simulink model "project_model_O10"  (R2025a)
settings: Solver=FixedStepAuto  StartTime=0.0  StopTime=10.0  FixedStep=1e-3  RelTol=1e-3  EnableMultiTasking=on
undefined symbols (not defined in the file): A0, A1, A2, A3, A4, D0, D10, D11, D12, D13, D2, D3, D4, D5, D6, D7, D8, D9, PTA0, PTA1, PTA2, PTB10, PTB11, PTB2, PTB23, PTB3, PTB9, PTC11, PTC16, PTC2, PTC3, PTC4, PTD0, PTD1, PTD2, PTD3
libraries: frdmk64flib x19
settings Model: ExtModeTrigDuration=5  Creator=justi  LastModifiedBy=justi
settings OptimizationCC: DefaultParameterBehavior=Inlined  EnhancedBackFolding=on  PassReuseOutputArgsAs=Individual arguments  ZeroExternalMemoryAtStartup=off  ZeroInternalMemoryAtStartup=off  MaxStackSize=64  OptimizeBlockOrder=speed  DifferentSizesBufferReuse=on  OptimizationCustomize=off  EfficientTunableParamExpr=on
settings DebuggingCC: ParameterTunabilityLossMsg=error
settings HardwareCC: ProdBitPerPointer=32.0  ProdBitPerSizeT=32.0  ProdBitPerPtrDiffT=32.0  ProdLargestAtomicInteger=Long  ProdLargestAtomicFloat=Double  ProdWordSize=32.0  ProdHWDeviceType=ARM Compatible->ARM Cortex
settings SFSimCC: MATLABDynamicMemAlloc=off
settings RTWCC: SystemTargetFile=ert.tlc  HardwareBoard=NXP FRDM-K64F  TLCOptions="-aInlineSetEventsForThisBaseRateFcn=TLC_FALSE -aSuppressMultiTaskScheduler=TLC_FALSE  -aRateBasedStepFcn=0"  TemplateMakefile=ert_default_tmf  Toolchain=GNU Tools for ARM Embedded Processors  Description=Embedded Coder
settings CodeAppCC: ForceParamTrailComments=on  IgnoreCustomStorageClasses=off  OperatorAnnotations=on  SimulinkDataObjDesc=on  SFDataObjDesc=on  InsertBlockDesc=on
settings ERTTargetCC: ExtModeTransport=4.0  ExtModeStaticAlloc=off  ExtModeMexFile=sendToCommService  ExtModeIntrfLevel=Level1

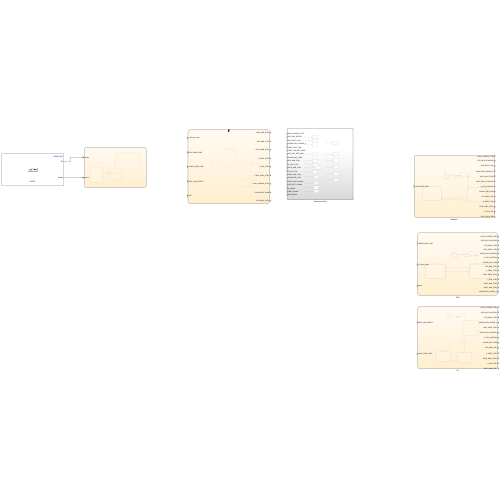
[thumbnail: Simulink's stored preview of the top-level diagram]
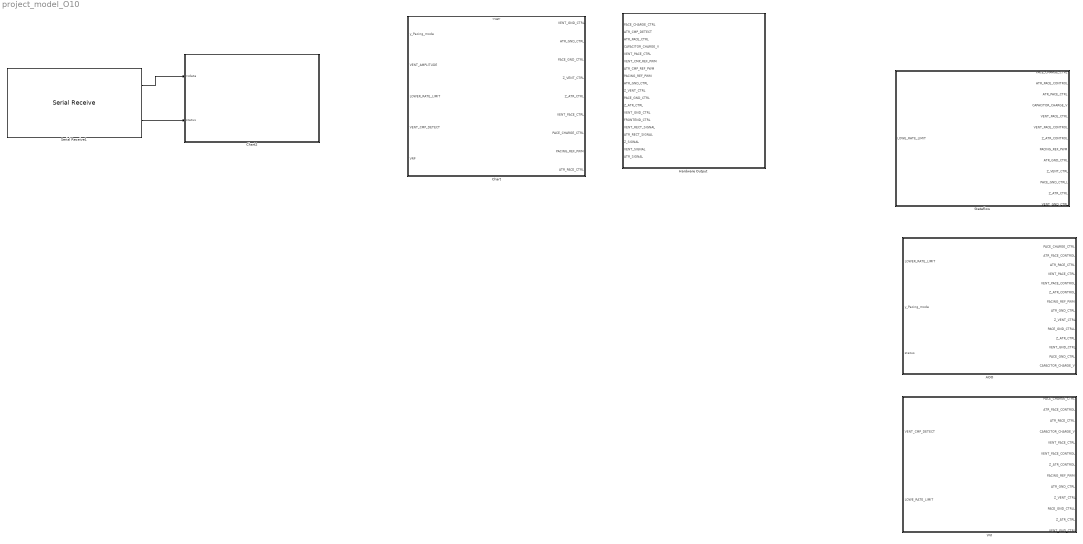
== system project_model_O10 ==
  AOO : Stateflow chart  TreatAsAtomicUnit=on
  Chart : Stateflow chart  TreatAsAtomicUnit=on
  Chart2 : Stateflow chart  TreatAsAtomicUnit=on
  Hardware Output : Subsystem
  Serial Receive1 : frdmk64flib/Serial Receive  SCIModule=0  Baudrate=uint32(9600)  Parity=None  StopBits=1  HardwareFlowControl=None  ByteOrder=LittleEndian  DataType=uint8  DataLength=10  BlockingMode=off  OutputStatus=on  SampleTime=0.1
  "Stateflow " : Stateflow chart  TreatAsAtomicUnit=on
  VVI : Stateflow chart  TreatAsAtomicUnit=on
  wires:
  Serial Receive1/2 -> Chart2/2(status)
  Serial Receive1/1 -> Chart2/1(rxdata)

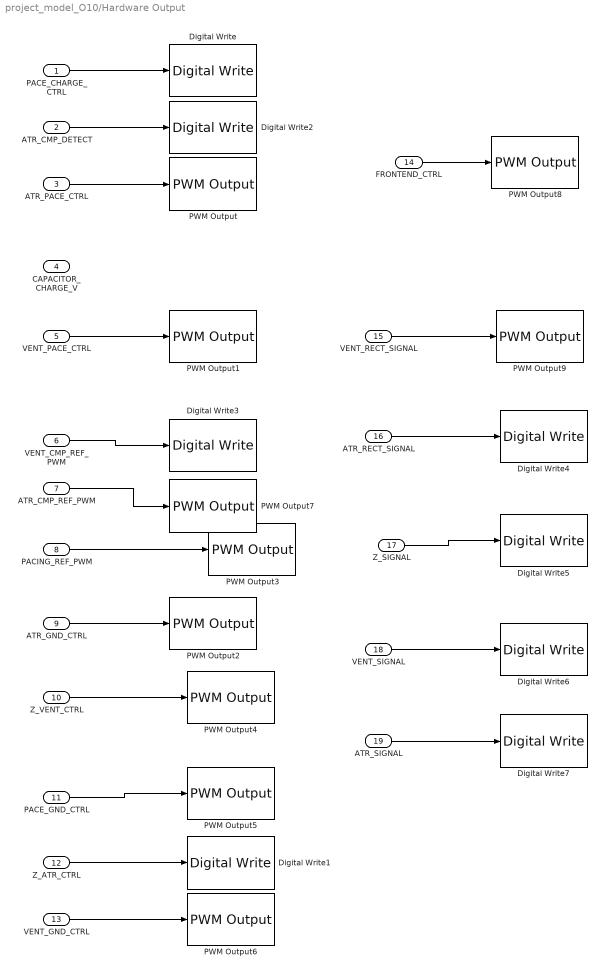
== system project_model_O10/Hardware Output ==
  PACE_CHARGE_CTRL : Inport
  ATR_CMP_DETECT : Inport  Port=2
  ATR_PACE_CTRL : Inport  Port=3
  CAPACITOR_CHARGE_V : Inport  Port=4
  VENT_PACE_CTRL : Inport  Port=5
  VENT_CMP_REF_PWM : Inport  Port=6
  ATR_CMP_REF_PWM : Inport  Port=7
  PACING_REF_PWM : Inport  Port=8
  ATR_GND_CTRL : Inport  Port=9
  Z_VENT_CTRL : Inport  Port=10
  PACE_GND_CTRL : Inport  Port=11
  Z_ATR_CTRL : Inport  Port=12
  VENT_GND_CTRL : Inport  Port=13
  FRONTEND_CTRL : Inport  Port=14
  VENT_RECT_SIGNAL : Inport  Port=15
  ATR_RECT_SIGNAL : Inport  Port=16
  Z_SIGNAL : Inport  Port=17
  VENT_SIGNAL : Inport  Port=18
  ATR_SIGNAL : Inport  Port=19
  Digital Write : frdmk64flib/Digital Write  Whichpin=PTB9 (D2)
  Digital Write1 : frdmk64flib/Digital Write  Whichpin=PTB23 (D4)
  Digital Write2 : frdmk64flib/Digital Write  Whichpin=PTC16 (D0)
  Digital Write3 : frdmk64flib/Digital Write  Whichpin=PTA1 (D3)
  Digital Write4 : frdmk64flib/Digital Write  Whichpin=PTB11 (A3)
  Digital Write5 : frdmk64flib/Digital Write  Whichpin=PTB10 (A2)
  Digital Write6 : frdmk64flib/Digital Write  Whichpin=PTB3 (A1)
  Digital Write7 : frdmk64flib/Digital Write  Whichpin=PTB2 (A0)
  PWM Output : frdmk64flib/PWM Output  Whichpin=PTA0 (D8)  InitialFrequency=2000  InitialDutyCycle=0
  PWM Output1 : frdmk64flib/PWM Output  Whichpin=PTC4 (D9)  InitialFrequency=2000  InitialDutyCycle=0
  PWM Output2 : frdmk64flib/PWM Output  Whichpin=PTD2 (D11)  InitialFrequency=2000  InitialDutyCycle=0
  PWM Output3 : frdmk64flib/PWM Output  Whichpin=PTA2 (D5)  InitialFrequency=2000  InitialDutyCycle=0
  PWM Output4 : frdmk64flib/PWM Output  Whichpin=PTC3 (D7)  InitialFrequency=2000  InitialDutyCycle=0
  PWM Output5 : frdmk64flib/PWM Output  Whichpin=PTD0 (D10)  InitialFrequency=2000  InitialDutyCycle=0
  PWM Output6 : frdmk64flib/PWM Output  Whichpin=PTD3 (D12)  InitialFrequency=2000  InitialDutyCycle=0
  PWM Output7 : frdmk64flib/PWM Output  Whichpin=PTC2 (D6)  InitialFrequency=2000  InitialDutyCycle=0
  PWM Output8 : frdmk64flib/PWM Output  Whichpin=PTD1 (D13)  InitialFrequency=2000  InitialDutyCycle=0
  PWM Output9 : frdmk64flib/PWM Output  Whichpin=PTC11 (A4)  InitialFrequency=2000  InitialDutyCycle=0
  wires:
  PACE_CHARGE_CTRL/1 -> Digital Write/1
  ATR_PACE_CTRL/1 -> PWM Output/1
  VENT_PACE_CTRL/1 -> PWM Output1/1
  ATR_GND_CTRL/1 -> PWM Output2/1
  PACING_REF_PWM/1 -> PWM Output3/1
  Z_VENT_CTRL/1 -> PWM Output4/1
  PACE_GND_CTRL/1 -> PWM Output5/1
  VENT_GND_CTRL/1 -> PWM Output6/1
  Z_ATR_CTRL/1 -> Digital Write1/1
  ATR_CMP_DETECT/1 -> Digital Write2/1
  VENT_CMP_REF_PWM/1 -> Digital Write3/1
  ATR_CMP_REF_PWM/1 -> PWM Output7/1
  FRONTEND_CTRL/1 -> PWM Output8/1
  VENT_RECT_SIGNAL/1 -> PWM Output9/1
  ATR_RECT_SIGNAL/1 -> Digital Write4/1
  Z_SIGNAL/1 -> Digital Write5/1
  VENT_SIGNAL/1 -> Digital Write6/1
  ATR_SIGNAL/1 -> Digital Write7/1

== stateflow chart project_model_O10/VVI ==
  state INITIAL
    entry:
  state STANDBY
  state Initial_Charge_Discharge
    PACE_GND_CTRL=1;
    VENT_PACE_CTRL=0;
    Z_ATR_CTRL=0;
    Z_VENT_CTRL=0;
    ATR_PACE_CTRL=0;
    ATR_GND_CTRL=0;
    VENT_GND_CTRL=1;
    ATR_PACE_CTRL=0;
    VENT_PACE_CTRL=0;
    PACING_REF_PWM=VENT_AMPLITUDE/5000;
    CAPACITOR_CHARGE_V=5;
    PACE_CHARGE_CTRL=1;
    PACE_CHARGE_CTRL=0;
    PACE_GND_CTRL=1;
    ATR_PACE_CTRL=0;
    ATR_GND_CTRL=0;
    Z_ATR_CTRL=0;
    Z_VENT_CTRL=0;
    VENT_GND_CTRL=0;
    VENT_PACE_CTRL=1;
  state Wait_State
  state Discharge
    PACE_CHARGE_CTRL=0;
    PACE_GND_CTRL=1;
    ATR_PACE_CTRL=0;
    ATR_GND_CTRL=0;
    Z_ATR_CTRL=0;
    Z_VENT_CTRL=0;
    VENT_GND_CTRL=0;
    VENT_PACE_CTRL=1;
  state Charge
    PACE_GND_CTRL=1;
    VENT_PACE_CTRL=0;
    Z_ATR_CTRL=0;
    Z_VENT_CTRL=0;
    ATR_PACE_CTRL=0;
    ATR_GND_CTRL=0;
    VENT_GND_CTRL=1;
    ATR_PACE_CTRL=0;
    VENT_PACE_CTRL=0;
    PACING_REF_PWM=VENT_AMPLITUDE/5000;
    CAPACITOR_CHARGE_V=5;
    PACE_CHARGE_CTRL=1;
  (default) -> INITIAL
  (junction 40) -> STANDBY [order 2]
  INITIAL -> STANDBY
  STANDBY -> (junction 40) : [status==0]
  (junction 40) -> Initial_Charge_Discharge [order 1] : [y_Pacing_mode == "VVI"]
  Initial_Charge_Discharge -> Wait_State
  Discharge -> Wait_State
  (junction 64) -> Wait_State [order 1] : [VENT_CMP_DETECT == true]
  Wait_State -> (junction 64) : [after(VRP, mSec)]
  (junction 64) -> Charge [order 2]
  Charge -> Discharge
  data: VENT_CMP_DETECT input; PACE_CHARGE_CTRL output; ATR_PACE_CONTROL output; ATR_PACE_CTRL output; CAPACITOR_CHARGE_V output; VENT_PACE_CTRL output; VENT_PACE_CONTROL output; Z_ATR_CONTROL output; PACING_REF_PWM output; ATR_GND_CTRL output; Z_VENT_CTRL output; PACE_GND_CTRLL output; Z_ATR_CTRL output; VENT_GND_CTRL output; LOWE_RATE_LIMIT input

== stateflow chart project_model_O10/Stateflow  ==
  state INITIAL
    entry:
  state STANDBY
  state Discharge
    PACE_CHARGE_CTRL=0;
    PACE_GND_CTRL=1;
    ATR_PACE_CTRL=0;
    ATR_GND_CTRL=0;
    Z_ATR_CTRL=0;
    Z_VENT_CTRL=0;
    VENT_GND_CTRL=0;
    VENT_PACE_CTRL=1;
  state Charge
    PACE_GND_CTRL=1;
    VENT_PACE_CTRL=0;
    Z_ATR_CTRL=0;
    Z_VENT_CTRL=0;
    ATR_PACE_CTRL=0;
    ATR_GND_CTRL=0;
    VENT_GND_CTRL=1;
    ATR_PACE_CTRL=0;
    VENT_PACE_CTRL=0;
    PACING_REF_PWM=2000;%todo
    CAPACITOR_CHARGE_V=5;
    PACE_CHARGE_CTRL=1;
  (default) -> INITIAL
  (junction 40) -> STANDBY [order 1]
  INITIAL -> STANDBY
  STANDBY -> (junction 40) : [status==0]
  (junction 40) -> Charge [order 2] : [y_Pacing_mode == "VOO"]
  Charge -> Discharge : [after((LOWER_RATE_LIMIT/2),sec)]
  Discharge -> Charge : [after((LOWER_RATE_LIMIT/2),sec)]
  data: PACE_CHARGE_CTRL output; ATR_PACE_CONTROL output; ATR_PACE_CTRL output; CAPACITOR_CHARGE_V output; VENT_PACE_CTRL output; VENT_PACE_CONTROL output; Z_ATR_CONTROL output; PACING_REF_PWM output; ATR_GND_CTRL output; Z_VENT_CTRL output; PACE_GND_CTRLL output; Z_ATR_CTRL output; VENT_GND_CTRL output; LOWE_RATE_LIMIT input

== stateflow chart project_model_O10/Chart ==
  state INITIAL3
    entry:
  state STANDBY3
  state Initial_Pace_VVI
    PACE_GND_CTRL=1;
    VENT_PACE_CTRL=0;
    Z_ATR_CTRL=0;
    Z_VENT_CTRL=0;
    ATR_PACE_CTRL=0;
    ATR_GND_CTRL=0;
    VENT_GND_CTRL=1;
    ATR_PACE_CTRL=0;
    VENT_PACE_CTRL=0;
    PACING_REF_PWM=VENT_AMPLITUDE/5000;
    CAPACITOR_CHARGE_V=5;
    PACE_CHARGE_CTRL=1;
    PACE_CHARGE_CTRL=0;
    PACE_GND_CTRL=1;
    ATR_PACE_CTRL=0;
    ATR_GND_CTRL=0;
    Z_ATR_CTRL=0;
    Z_VENT_CTRL=0;
    VENT_GND_CTRL=0;
    VENT_PACE_CTRL=1;
  state Discharge_VOO
    PACE_CHARGE_CTRL=0;
    PACE_GND_CTRL=1;
    ATR_PACE_CTRL=0;
    ATR_GND_CTRL=0;
    Z_ATR_CTRL=0;
    Z_VENT_CTRL=0;
    VENT_GND_CTRL=0;
    VENT_PACE_CTRL=1;
  state Charge_VOO
    PACE_GND_CTRL=1;
    VENT_PACE_CTRL=0;
    Z_ATR_CTRL=0;
    Z_VENT_CTRL=0;
    ATR_PACE_CTRL=0;
    ATR_GND_CTRL=0;
    VENT_GND_CTRL=1;
    ATR_PACE_CTRL=0;
    VENT_PACE_CTRL=0;
    PACING_REF_PWM=VENT_AMPLITUDE/5000;
    PACE_CHARGE_CTRL=1;
  state Discharge_AOO
    PACE_CHARGE_CTRL=0;
    PACE_GND_CTRL=1;
    VENT_PACE_CTRL=0;
    VENT_GND_CTRL=0;
    Z_VENT_CTRL=0;
    Z_ATR_CTRL=0;
    ATR_GND_CTRL=0;
    ATR_PACE_CTRL=1;
  state Charge_AOO
    PACE_GND_CTRL=1;
    ATR_PACE_CTRL=0;
    Z_VENT_CTRL=0;
    Z_ATR_CTRL=0;
    VENT_PACE_CTRL=0;
    VENT_GND_CTRL=0;
    ATR_GND_CTRL=1;
    VENT_PACE_CTRL=0;
    ATR_PACE_CTRL=0;
    PACING_REF_PWM=2000;%todo
    PACE_CHARGE_CTRL=1;
  state Wait_State
  state Discharge_VVI
    PACE_CHARGE_CTRL=0;
    PACE_GND_CTRL=1;
    ATR_PACE_CTRL=0;
    ATR_GND_CTRL=0;
    Z_ATR_CTRL=0;
    Z_VENT_CTRL=0;
    VENT_GND_CTRL=0;
    VENT_PACE_CTRL=1;
  state Charge_VVI
    PACE_GND_CTRL=1;
    VENT_PACE_CTRL=0;
    Z_ATR_CTRL=0;
    Z_VENT_CTRL=0;
    ATR_PACE_CTRL=0;
    ATR_GND_CTRL=0;
    VENT_GND_CTRL=1;
    ATR_PACE_CTRL=0;
    VENT_PACE_CTRL=0;
    PACING_REF_PWM=VENT_AMPLITUDE/5000;
    CAPACITOR_CHARGE_V=5;
    PACE_CHARGE_CTRL=1;
  (default) -> INITIAL3
  (junction 57) -> STANDBY3 [order 4]
  INITIAL3 -> STANDBY3
  STANDBY3 -> (junction 57) : [status==0]
  (junction 57) -> Initial_Pace_VVI [order 1] : [y_Pacing_mode == "VVI"]
  (junction 57) -> Charge_VOO [order 3] : [y_Pacing_mode == "VOO"]
  (junction 57) -> Charge_AOO [order 2] : [y_Pacing_mode == "AOO"]
  Charge_AOO -> Discharge_AOO : [after((LOWER_RATE_LIMIT/2),mSec)]
  Discharge_AOO -> Charge_AOO : [after((LOWER_RATE_LIMIT/2),mSec)]
  Charge_VOO -> Discharge_VOO : [after((LOWER_RATE_LIMIT/2),mSec)]
  Discharge_VOO -> Charge_VOO : [after((LOWER_RATE_LIMIT/2),mSec)]
  Initial_Pace_VVI -> Wait_State
  Discharge_VVI -> Wait_State
  (junction 28) -> Wait_State [order 1] : [VENT_CMP_DETECT == true]
  Wait_State -> (junction 28) : [after(VRP, mSec)]
  (junction 28) -> Charge_VVI [order 2] : [after(LOWER_RATE_LIMIT-VRP, mSec)]
  Charge_VVI -> Discharge_VVI
  data: y_Pacing_mode input; VENT_GND_CTRL output; ATR_GND_CTRL output; PACE_GND_CTRL output; Z_VENT_CTRL output; Z_ATR_CTRL output; VENT_PACE_CTRL output; PACE_CHARGE_CTRL output; PACING_REF_PWM output; ATR_PACE_CTRL output; VENT_AMPLITUDE input; LOWER_RATE_LIMIT input; VENT_CMP_DETECT input; VRP input
  events: mSec input RISING_EDGE_EVENT

== stateflow chart project_model_O10/Chart2 ==
  state SET_PARAM_
    entry:
    LOWER_RATE_LIMIT=typecast(rxdata(3:4),'uint16');
    UPPER_RATE_LIMIT=typecast(rxdata(5:6),'uint16');
    MAXIMUM_SENSOR_RATE=typecast(rxdata(7:8),'uint16');
    FIXED_AV_DELAY=typecast(rxdata(9:10),'uint16');
    DYNAMIC_AV_DELAY=typecast(rxdata(11:12),'uint16');
    SENSED_AV_DELAY_OFFSET=typecast(rxdata(13:14),'uint16');
    ATRIAL_AMPLITUDE=typecast(rxdata(15:16),'uint16');
    VENTRICULAR_AMPLITUDE=typecast(rxdata(17:18),'uint16');
    ATRIAL_PULSE_WIDTH=typecast(rxdata(19:20),'uint16');
    VENTRICULAR_PULSE_WIDTH=typecast(rxdata(21:22),'uint16');
    ATRIAL_SENSITIVITY=typecast(rxdata(23:24),'uint16');
    VENTRICULAR_SENSITIVITY=typecast(rxdata(25:26),'uint16');
    VRP=typecast(rxdata(27:28),'uint16');
    ARP=typecast(rxdata(29:30),'uint16');
    PVARP=typecast(rxdata(31:32),'uint16');
    PVARP_EXTENSION=typecast(rxdata(33:34),'uint16');
    HYSTERESIS=typecast(rxdata(35:36),'uint16');
    RATE_SMOOTHING=typecast(rxdata(37:38),'uint16');
    ATR_DURATION=typecast(rxdata(39:40),'uint16');
    ATR_FALLBACK_MODE=typecast(rxdata(41:42),'uint16');
    ATR_FALLBACK_TIME=typecast(rxdata(43:44),'uint16');
    ACTIVITY_THRESHOLD=typecast(rxdata(45:46),'uint16');
    REACTION_TIME=typecast(rxdata(47:48),'uint16');
    RESPONSE_FACTOR=typecast(rxdata(49:50),'uint16');
    RECOVERY_TIME=typecast(rxdata(51:52),'uint16');
  state INITIAL
    entry:
    LOWER_RATE_LIMIT = 0;
    UPPER_RATE_LIMIT = 0;
    MAXIMUM_SENSOR_RATE = 0;
    FIXED_AV_DELAY = 0;
    DYNAMIC_AV_DELAY = 0;
    SENSED_AV_DELAY_OFFSET = 0;
    ATRIAL_AMPLITUDE = 0;
    VENTRICULAR_AMPLITUDE = 0;
    ATRIAL_PULSE_WIDTH = 0;
    VENTRICULAR_PULSE_WIDTH = 0;
    ATRIAL_SENSITIVITY = 0;
    VENTRICULAR_SENSITIVITY = 0;
    VRP = 0; ARP = 0; PVARP = 0;
    PVARP_EXTENSION = 0;
    HYSTERESIS = 0;
    RATE_SMOOTHING = 0;
    ATR_DURATION = 0;
    ATR_FALLBACK_MODE = 0;
    ATR_FALLBACK_TIME = 0;
    ACTIVITY_THRESHOLD = 0;
    REACTION_TIME = 0;
    RESPONSE_FACTOR = 0;
    RECOVERY_TIME = 0;
  state STANDBY
    %Wait for COM
  state ECHO_PARAM
    entry:
    send_params();
  SET_PARAM_ -> STANDBY
  (default) -> INITIAL
  (junction 10) -> SET_PARAM_ [order 1] : [rx_data (2) == hex2dec('55')]
  (junction 8) -> STANDBY [order 2]
  INITIAL -> STANDBY
  STANDBY -> (junction 8) : [status == 0]
  (junction 8) -> (junction 10) [order 1] : [rx_data (1) == hex2dec('16')]
  (junction 10) -> ECHO_PARAM [order 2] : [rx_data (2) == hex2dec('22')]
  ECHO_PARAM -> STANDBY
  data: rxdata input; status input

== stateflow chart project_model_O10/AOO ==
  state INITIAL
    entry:
  state STANDBY
  state Discharge
    PACE_CHARGE_CTRL=0;
    PACE_GND_CTRL=1;
    VENT_PACE_CTRL=0;
    VENT_GND_CTRL=0;
    Z_VENT_CTRL=0;
    Z_ATR_CTRL=0;
    ATR_GND_CTRL=0;
    ATR_PACE_CTRL=1;
  state Charge
    PACE_GND_CTRL=1;
    ATR_PACE_CTRL=0;
    Z_VENT_CTRL=0;
    Z_ATR_CTRL=0;
    VENT_PACE_CTRL=0;
    VENT_GND_CTRL=0;
    ATR_GND_CTRL=1;
    VENT_PACE_CTRL=0;
    ATR_PACE_CTRL=0;
    PACING_REF_PWM=2000;%todo
    CAPACITOR_CHARGE_V=5;
    PACE_CHARGE_CTRL=1;
  (default) -> INITIAL
  (junction 35) -> STANDBY [order 2]
  INITIAL -> STANDBY
  STANDBY -> (junction 35) : [status==0]
  (junction 35) -> Charge [order 1] : [y_Pacing_mode == "AOO"]
  Charge -> Discharge : [after((LOWER_RATE_LIMIT/2),sec)]
  Discharge -> Charge : [after((LOWER_RATE_LIMIT/2),sec)]
  data: PACE_CHARGE_CTRL output; ATR_PACE_CONTROL output; ATR_PACE_CTRL output; VENT_PACE_CTRL output; VENT_PACE_CONTROL output; Z_ATR_CONTROL output; PACING_REF_PWM output; ATR_GND_CTRL output; Z_VENT_CTRL output; PACE_GND_CTRLL output; Z_ATR_CTRL output; VENT_GND_CTRL output; PACE_GND_CTRL output; LOWER_RATE_LIMIT input; y_Pacing_mode input; status input; CAPACITOR_CHARGE_V output
